simulink model "SwitchCase"  (Simulink 9.0)
settings: Solver=FixedStepDiscrete  StartTime=0.0  StopTime=1  FixedStep=0.020000  MaxStep=1  RelTol=1e-3  EnableMultiTasking=on
model workspace (MAT data in the model file):
  input_struct.time = [0; 0.02; 0.04; 0.06; 0.08; 0.1; 0.12; 0.14; 0.16; 0.18; 0.2; 0.22; 0.24; 0.26; 0.28; 0.3; 0.32; 0.34; 0.36; 0.38; 0.4; 0.42; 0.44; 0.46; 0.48; 0.5; 0.52; 0.54; 0.56; 0.58; 0.6; 0.62; 0.64; 0.66; 0.68; 0.7; 0.72; 0.74; 0.76; 0.78; 0.8; 0.82; 0.84; 0.86; 0.88; 0.9; 0.92; 0.94; 0.96; 0.98; 1; 1.02; 1.04; 1.06; 1.08; 1.1; 1.12; 1.14; 1.16; 1.18; 1.2; 1.22; 1.24; 1.26; 1.28; 1.3; 1.32; 1.34; 1.36; 1.38; 1.4; 1.42; 1.44; 1.46; 1.48; 1.5; 1.52; 1.54; 1.56; 1.58; 1.6; 1.62; 1.64; 1.66; 1.68; 1.7; 1.72; 1.74; 1.76; 1.78; 1.8; 1.82; 1.84; 1.86; 1.88; 1.9; 1.92; 1.94; 1.96; 1.98]
  input_struct.signals(1).name = 'In1'
  input_struct.signals(1).values = [41.8890583008; 98.5239618563; 86.4389740185; -81.5541007222; 90.7079945659; -67.4408682365; 94.0910174544; 19.4013330536; -51.9545761753; -85.9409677044; -39.9917569782; 62.7089647794; -84.6580251598; -29.1053809122; -73.5978251182; -68.3640739331; -87.5705896765; 40.3686957785; -82.7036605841; 23.3574479124; -65.2456833551; 30.2802129477; -0.260718803377; -43.0978622866; 66.1119477471; 63.6719764967; 87.6338807507; -99.934780732; 28.0778449268; -98.5288614447; -78.7157786615; -78.641117349; -26.5781912292; -52.0784598827; -30.7719596605; -50.07603292; -22.5871371712; -15.7923259133; 28.0154578291; 57.5105945913; -46.0011152759; 68.7964721452; 48.0936760444; 65.2203897828; -63.561550525; -86.9127634489; 22.0700524226; 40.310561855; -77.6764574494; -80.835253506; 19.5667544642; 62.446522071; 62.9156348073; -82.1126069713; 46.2557410651; 80.7713152448; -9.5536425569; -85.8624647283; -51.7443689865; 46.3730119647; -91.9016768682; -15.0954474287; 8.04301740858; 90.7655675788; -58.2188516021; -76.7335807551; 29.2440135786; -78.317782043; 96.6993848433; -50.3311923108; 21.2711440264; 63.3390545561; 66.0108425214; -2.19213350976; 52.1456512236; 83.0215870698; 80.1949912529; -57.1524979853; 9.41222119564; 56.9418961991; -61.1117811496; 49.3778303995; -4.88835511173; 16.6517162455; -47.8903836296; -83.0355080738; -40.3734297632; 83.4258717754; -5.8963614508; -46.1064893531; 52.594095389; 54.4344210366; -95.7400751781; 75.9972384995; 59.6340368275; -35.1669522901; 33.8088833278; -40.7412273298; 85.9904087354; -43.6079130171]
  input_struct.signals(1).dimensions = 1
  input_struct.signals(2).name = 'In7'
  input_struct.signals(2).values = [0; 1; 0; 1; 1; 0; 0; 1; 0; 1; 0; 0; 0; 1; 0; 0; 1; 1; 1; 0; 0; 1; 0; 0; 1; 1; 0; 1; 0; 1; 0; 0; 1; 0; 0; 1; 0; 0; 1; 0; 0; 0; 0; 0; 0; 1; 1; 0; 0; 1; 1; 1; 1; 0; 1; 0; 0; 0; 1; 0; 1; 1; 0; 1; 1; 1; 0; 0; 1; 1; 0; 1; 0; 1; 0; 1; 1; 0; 0; 0; 1; 1; 1; 1; 0; 1; 1; 0; 1; 0; 0; 0; 1; 1; 1; 0; 0; 0; 0; 1]
  input_struct.signals(2).dimensions = 1
  input_struct.signals(3).name = 'In2'
  input_struct.signals(3).values = [-73.8696805284; -89.7288534639; 25.5012953943; -94.1824896299; -72.761078071; 38.9111197379; 3.13579149085; 8.51648406295; 61.6967017939; 58.737205938; 0.373417407607; -44.6735884264; -76.0670117794; 77.3195520316; 94.0577982224; 88.5052625756; 27.6256265025; -81.8819695917; -85.0583770202; -63.5098127598; -93.6624675996; 44.9872616092; -71.1682380107; 27.1853633216; 57.969511737; 13.2506253218; -24.5172152223; 64.3172231023; -39.0238340987; -36.1253804926; 56.9959782766; 0.747287411455; -47.8006536133; 46.4951048313; -67.4100069963; 84.2150444204; -55.555307467; -83.2782565304; -85.2596892516; 53.9103315324; 63.5354053389; 48.0851070561; 51.6497574356; 92.2389960221; -6.71500758009; 57.3992976002; -15.4863832646; 88.7459916859; -99.7371204024; 96.2535814309; 14.0388364617; -30.7058891183; 11.5006106218; -40.0430594997; -68.1854354949; 33.0512571745; 36.840556655; 58.4818724697; -30.275112468; -49.9850533294; -30.9993229412; -34.2734814269; 85.4971065784; 51.2144864907; -42.3522733151; 21.2359752297; 53.2058728474; 69.230468855; 80.3962383758; 19.1414295158; -86.2927710768; -56.3913250112; 73.8816983075; -17.1564291701; 32.2418304003; 56.6969680644; -50.4227984754; 10.8850577706; -54.0829209729; -98.6174472059; 53.3278794469; -95.6333500971; -21.3793130789; -49.4919688486; -59.1566157212; 32.4558934433; 82.948416006; -98.6194904513; 49.2846400724; 59.9341588339; 81.5597882142; 94.9147870771; -76.0273017736; 3.79395268337; 64.3949623376; 27.4045597486; 90.7820753799; 89.3852746454; 93.3210490664; -86.5311623056]
  input_struct.signals(3).dimensions = 1
settings Model: SuppressorTable=22 serialization::archive 11 0 6 0 0 0 0 0  Creator=arnaud  LastModifiedBy=hbourbou
settings DataIOCC: LimitDataPoints=on  SaveFormat=Structure
settings DebuggingCC: UnderspecifiedInitializationDetection=Simplified  MergeDetectMultiDrivingBlocksExec=error  SolverPrmCheckMsg=warning
settings GRTTargetCC: GeneratePreprocessorConditionals=Disable all
settings ConfigComp: CovSFcnEnable=off

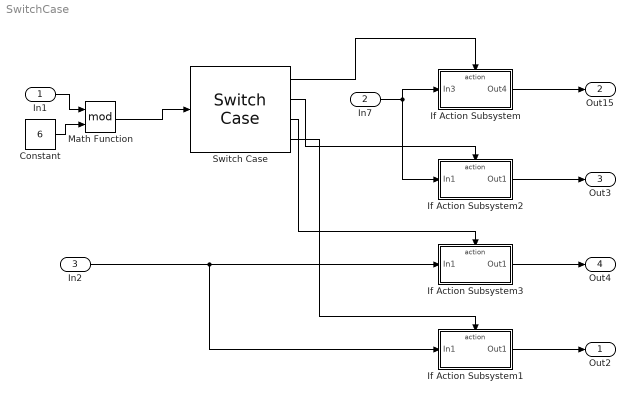
== system SwitchCase ==
  In1 : Inport  OutDataTypeStr=int8
  In7 : Inport  Port=2  OutDataTypeStr=boolean
  In2 : Inport  Port=3  OutDataTypeStr=double
  Constant : Constant  Value=6  OutDataTypeStr=int8
  If Action Subsystem : Subsystem  TreatAsAtomicUnit=on
      settings: MinAlgLoopOccurrences=on
  If Action Subsystem1 : Subsystem  TreatAsAtomicUnit=on
      settings: MinAlgLoopOccurrences=on
  If Action Subsystem2 : Subsystem  TreatAsAtomicUnit=on
      settings: MinAlgLoopOccurrences=on
  If Action Subsystem3 : Subsystem  TreatAsAtomicUnit=on
      settings: MinAlgLoopOccurrences=on
  Math Function : Math  Operator=mod  SaturateOnIntegerOverflow=on
  Switch Case : SwitchCase  CaseConditions={1,2,[3 6],4}  ShowDefaultCase=off
  Out2 : Outport
  Out15 : Outport  Port=2
  Out3 : Outport  Port=3
  Out4 : Outport  Port=4
  wires:
  In1/1 -> Math Function/1
  Switch Case/1 -> If Action Subsystem/Action
  Switch Case/4 -> If Action Subsystem1/Action
  If Action Subsystem1/1(Out1) -> Out2/1
  In7/1 -> If Action Subsystem2/1(In1), If Action Subsystem/1(In3)
  If Action Subsystem/1(Out4) -> Out15/1
  If Action Subsystem2/1(Out1) -> Out3/1
  If Action Subsystem3/1(Out1) -> Out4/1
  Switch Case/3 -> If Action Subsystem3/Action
  Switch Case/2 -> If Action Subsystem2/Action
  In2/1 -> If Action Subsystem1/1(In1), If Action Subsystem3/1(In1)
  Math Function/1 -> Switch Case/1
  Constant/1 -> Math Function/2

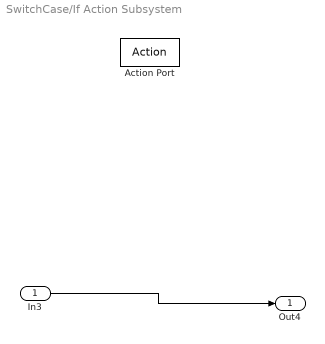
== system SwitchCase/If Action Subsystem ==
  In3 : Inport  OutDataTypeStr=boolean
  Action Port : ActionPort  ActionType=case
  Out4 : Outport
  wires:
  In3/1 -> Out4/1

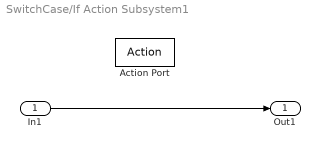
== system SwitchCase/If Action Subsystem1 ==
  In1 : Inport  OutDataTypeStr=double
  Action Port : ActionPort  ActionType=case
  Out1 : Outport
  wires:
  In1/1 -> Out1/1

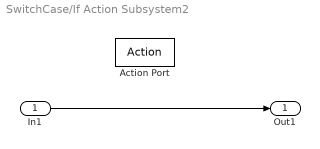
== system SwitchCase/If Action Subsystem2 ==
  In1 : Inport  OutDataTypeStr=boolean
  Action Port : ActionPort  ActionType=case
  Out1 : Outport
  wires:
  In1/1 -> Out1/1

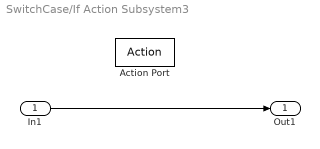
== system SwitchCase/If Action Subsystem3 ==
  In1 : Inport  OutDataTypeStr=double
  Action Port : ActionPort  ActionType=case
  Out1 : Outport
  wires:
  In1/1 -> Out1/1
